simulink model "UZ_EnDat_be4_diffrework"  (R2023b)
settings: Solver=FixedStepDiscrete  StartTime=0  StopTime=0.002  RelTol=1e-3
model workspace (MAT data in the model file):
  Select = 0
libraries: hdlsllib x207, simulink x17, simulink_extras x3
(part 5 of 5)

== system UZ_EnDat_be4_diffrework/UZ_ENDAT/RESPONSESLICER5X/25BITSLICER/responseslicer2 ==
  DATA : Inport  OutDataTypeStr=uint64
  Bit Slice1 : hdlsllib/Logic and Bit Operations/Bit Slice  lidx=2  ridx=2
  Bit Slice3 : hdlsllib/Logic and Bit Operations/Bit Slice  lidx=31  ridx=27
  Bit Slice4 : hdlsllib/Logic and Bit Operations/Bit Slice  lidx=26  ridx=2
  Data Type Conversion1 : DataTypeConversion  OutDataTypeStr=boolean  SaturateOnIntegerOverflow=off  RndMeth=Floor
  Data Type Conversion3 : DataTypeConversion  OutDataTypeStr=uint8  SaturateOnIntegerOverflow=off  RndMeth=Floor
  Data Type Conversion4 : DataTypeConversion  OutDataTypeStr=uint32  SaturateOnIntegerOverflow=off  RndMeth=Floor
  Terminator : Terminator
  CRC : Outport  OutDataTypeStr=uint8
  payload : Outport  Port=2  OutDataTypeStr=uint32
  error : Outport  Port=3  OutDataTypeStr=boolean
  wires:
  DATA/1 -> Terminator/1, Bit Slice1/1, Bit Slice4/1, Bit Slice3/1
  Bit Slice3/1 -> Data Type Conversion3/1
  Bit Slice4/1 -> Data Type Conversion4/1
  Data Type Conversion3/1 -> CRC/1
  Data Type Conversion4/1 -> payload/1
  Bit Slice1/1 -> Data Type Conversion1/1
  Data Type Conversion1/1 -> error/1

== system UZ_EnDat_be4_diffrework/UZ_ENDAT/RESPONSESLICER5X/25BITSLICER/responseslicer3 ==
  DATA : Inport  OutDataTypeStr=uint64
  Bit Slice1 : hdlsllib/Logic and Bit Operations/Bit Slice  lidx=2  ridx=2
  Bit Slice3 : hdlsllib/Logic and Bit Operations/Bit Slice  lidx=31  ridx=27
  Bit Slice4 : hdlsllib/Logic and Bit Operations/Bit Slice  lidx=26  ridx=2
  Data Type Conversion1 : DataTypeConversion  OutDataTypeStr=boolean  SaturateOnIntegerOverflow=off  RndMeth=Floor
  Data Type Conversion3 : DataTypeConversion  OutDataTypeStr=uint8  SaturateOnIntegerOverflow=off  RndMeth=Floor
  Data Type Conversion4 : DataTypeConversion  OutDataTypeStr=uint32  SaturateOnIntegerOverflow=off  RndMeth=Floor
  Terminator : Terminator
  CRC : Outport  OutDataTypeStr=uint8
  payload : Outport  Port=2  OutDataTypeStr=uint32
  error : Outport  Port=3  OutDataTypeStr=boolean
  wires:
  DATA/1 -> Terminator/1, Bit Slice1/1, Bit Slice4/1, Bit Slice3/1
  Bit Slice3/1 -> Data Type Conversion3/1
  Bit Slice4/1 -> Data Type Conversion4/1
  Data Type Conversion3/1 -> CRC/1
  Data Type Conversion4/1 -> payload/1
  Bit Slice1/1 -> Data Type Conversion1/1
  Data Type Conversion1/1 -> error/1

== system UZ_EnDat_be4_diffrework/UZ_ENDAT/RESPONSESLICER5X/25BITSLICER/responseslicer4 ==
  DATA : Inport  OutDataTypeStr=uint64
  Bit Slice1 : hdlsllib/Logic and Bit Operations/Bit Slice  lidx=2  ridx=2
  Bit Slice3 : hdlsllib/Logic and Bit Operations/Bit Slice  lidx=31  ridx=27
  Bit Slice4 : hdlsllib/Logic and Bit Operations/Bit Slice  lidx=26  ridx=2
  Data Type Conversion1 : DataTypeConversion  OutDataTypeStr=boolean  SaturateOnIntegerOverflow=off  RndMeth=Floor
  Data Type Conversion3 : DataTypeConversion  OutDataTypeStr=uint8  SaturateOnIntegerOverflow=off  RndMeth=Floor
  Data Type Conversion4 : DataTypeConversion  OutDataTypeStr=uint32  SaturateOnIntegerOverflow=off  RndMeth=Floor
  Terminator : Terminator
  CRC : Outport  OutDataTypeStr=uint8
  payload : Outport  Port=2  OutDataTypeStr=uint32
  error : Outport  Port=3  OutDataTypeStr=boolean
  wires:
  DATA/1 -> Terminator/1, Bit Slice1/1, Bit Slice4/1, Bit Slice3/1
  Bit Slice3/1 -> Data Type Conversion3/1
  Bit Slice4/1 -> Data Type Conversion4/1
  Data Type Conversion3/1 -> CRC/1
  Data Type Conversion4/1 -> payload/1
  Bit Slice1/1 -> Data Type Conversion1/1
  Data Type Conversion1/1 -> error/1

== system UZ_EnDat_be4_diffrework/UZ_ENDAT/RESPONSESLICER5X/27BITSLICER/responseslicer ==
  DATA : Inport  OutDataTypeStr=uint64
  Bit Slice1 : hdlsllib/Logic and Bit Operations/Bit Slice  lidx=2  ridx=2
  Bit Slice3 : hdlsllib/Logic and Bit Operations/Bit Slice  lidx=33  ridx=29
  Bit Slice4 : hdlsllib/Logic and Bit Operations/Bit Slice  lidx=28  ridx=2
  Data Type Conversion1 : DataTypeConversion  OutDataTypeStr=boolean  SaturateOnIntegerOverflow=off  RndMeth=Floor
  Data Type Conversion3 : DataTypeConversion  OutDataTypeStr=uint8  SaturateOnIntegerOverflow=off  RndMeth=Floor
  Data Type Conversion4 : DataTypeConversion  OutDataTypeStr=uint32  SaturateOnIntegerOverflow=off  RndMeth=Floor
  Terminator : Terminator
  CRC : Outport  OutDataTypeStr=uint8
  payload : Outport  Port=2  OutDataTypeStr=uint32
  error : Outport  Port=3  OutDataTypeStr=boolean
  wires:
  DATA/1 -> Terminator/1, Bit Slice1/1, Bit Slice4/1, Bit Slice3/1
  Bit Slice3/1 -> Data Type Conversion3/1
  Bit Slice4/1 -> Data Type Conversion4/1
  Data Type Conversion3/1 -> CRC/1
  Data Type Conversion4/1 -> payload/1
  Bit Slice1/1 -> Data Type Conversion1/1
  Data Type Conversion1/1 -> error/1

== system UZ_EnDat_be4_diffrework/UZ_ENDAT/RESPONSESLICER5X/27BITSLICER/responseslicer1 ==
  DATA : Inport  OutDataTypeStr=uint64
  Bit Slice1 : hdlsllib/Logic and Bit Operations/Bit Slice  lidx=2  ridx=2
  Bit Slice3 : hdlsllib/Logic and Bit Operations/Bit Slice  lidx=33  ridx=29
  Bit Slice4 : hdlsllib/Logic and Bit Operations/Bit Slice  lidx=28  ridx=2
  Data Type Conversion1 : DataTypeConversion  OutDataTypeStr=boolean  SaturateOnIntegerOverflow=off  RndMeth=Floor
  Data Type Conversion3 : DataTypeConversion  OutDataTypeStr=uint8  SaturateOnIntegerOverflow=off  RndMeth=Floor
  Data Type Conversion4 : DataTypeConversion  OutDataTypeStr=uint32  SaturateOnIntegerOverflow=off  RndMeth=Floor
  Terminator : Terminator
  CRC : Outport  OutDataTypeStr=uint8
  payload : Outport  Port=2  OutDataTypeStr=uint32
  error : Outport  Port=3  OutDataTypeStr=boolean
  wires:
  DATA/1 -> Terminator/1, Bit Slice1/1, Bit Slice4/1, Bit Slice3/1
  Bit Slice3/1 -> Data Type Conversion3/1
  Bit Slice4/1 -> Data Type Conversion4/1
  Data Type Conversion3/1 -> CRC/1
  Data Type Conversion4/1 -> payload/1
  Bit Slice1/1 -> Data Type Conversion1/1
  Data Type Conversion1/1 -> error/1

== system UZ_EnDat_be4_diffrework/UZ_ENDAT/RESPONSESLICER5X/27BITSLICER/responseslicer2 ==
  DATA : Inport  OutDataTypeStr=uint64
  Bit Slice1 : hdlsllib/Logic and Bit Operations/Bit Slice  lidx=2  ridx=2
  Bit Slice3 : hdlsllib/Logic and Bit Operations/Bit Slice  lidx=33  ridx=29
  Bit Slice4 : hdlsllib/Logic and Bit Operations/Bit Slice  lidx=28  ridx=2
  Data Type Conversion1 : DataTypeConversion  OutDataTypeStr=boolean  SaturateOnIntegerOverflow=off  RndMeth=Floor
  Data Type Conversion3 : DataTypeConversion  OutDataTypeStr=uint8  SaturateOnIntegerOverflow=off  RndMeth=Floor
  Data Type Conversion4 : DataTypeConversion  OutDataTypeStr=uint32  SaturateOnIntegerOverflow=off  RndMeth=Floor
  Terminator : Terminator
  CRC : Outport  OutDataTypeStr=uint8
  payload : Outport  Port=2  OutDataTypeStr=uint32
  error : Outport  Port=3  OutDataTypeStr=boolean
  wires:
  DATA/1 -> Terminator/1, Bit Slice1/1, Bit Slice4/1, Bit Slice3/1
  Bit Slice3/1 -> Data Type Conversion3/1
  Bit Slice4/1 -> Data Type Conversion4/1
  Data Type Conversion3/1 -> CRC/1
  Data Type Conversion4/1 -> payload/1
  Bit Slice1/1 -> Data Type Conversion1/1
  Data Type Conversion1/1 -> error/1

== system UZ_EnDat_be4_diffrework/UZ_ENDAT/RESPONSESLICER5X/27BITSLICER/responseslicer3 ==
  DATA : Inport  OutDataTypeStr=uint64
  Bit Slice1 : hdlsllib/Logic and Bit Operations/Bit Slice  lidx=2  ridx=2
  Bit Slice3 : hdlsllib/Logic and Bit Operations/Bit Slice  lidx=33  ridx=29
  Bit Slice4 : hdlsllib/Logic and Bit Operations/Bit Slice  lidx=28  ridx=2
  Data Type Conversion1 : DataTypeConversion  OutDataTypeStr=boolean  SaturateOnIntegerOverflow=off  RndMeth=Floor
  Data Type Conversion3 : DataTypeConversion  OutDataTypeStr=uint8  SaturateOnIntegerOverflow=off  RndMeth=Floor
  Data Type Conversion4 : DataTypeConversion  OutDataTypeStr=uint32  SaturateOnIntegerOverflow=off  RndMeth=Floor
  Terminator : Terminator
  CRC : Outport  OutDataTypeStr=uint8
  payload : Outport  Port=2  OutDataTypeStr=uint32
  error : Outport  Port=3  OutDataTypeStr=boolean
  wires:
  DATA/1 -> Terminator/1, Bit Slice1/1, Bit Slice4/1, Bit Slice3/1
  Bit Slice3/1 -> Data Type Conversion3/1
  Bit Slice4/1 -> Data Type Conversion4/1
  Data Type Conversion3/1 -> CRC/1
  Data Type Conversion4/1 -> payload/1
  Bit Slice1/1 -> Data Type Conversion1/1
  Data Type Conversion1/1 -> error/1

== system UZ_EnDat_be4_diffrework/UZ_ENDAT/RESPONSESLICER5X/27BITSLICER/responseslicer4 ==
  DATA : Inport  OutDataTypeStr=uint64
  Bit Slice1 : hdlsllib/Logic and Bit Operations/Bit Slice  lidx=2  ridx=2
  Bit Slice3 : hdlsllib/Logic and Bit Operations/Bit Slice  lidx=33  ridx=29
  Bit Slice4 : hdlsllib/Logic and Bit Operations/Bit Slice  lidx=28  ridx=2
  Data Type Conversion1 : DataTypeConversion  OutDataTypeStr=boolean  SaturateOnIntegerOverflow=off  RndMeth=Floor
  Data Type Conversion3 : DataTypeConversion  OutDataTypeStr=uint8  SaturateOnIntegerOverflow=off  RndMeth=Floor
  Data Type Conversion4 : DataTypeConversion  OutDataTypeStr=uint32  SaturateOnIntegerOverflow=off  RndMeth=Floor
  Terminator : Terminator
  CRC : Outport  OutDataTypeStr=uint8
  payload : Outport  Port=2  OutDataTypeStr=uint32
  error : Outport  Port=3  OutDataTypeStr=boolean
  wires:
  DATA/1 -> Terminator/1, Bit Slice1/1, Bit Slice4/1, Bit Slice3/1
  Bit Slice3/1 -> Data Type Conversion3/1
  Bit Slice4/1 -> Data Type Conversion4/1
  Data Type Conversion3/1 -> CRC/1
  Data Type Conversion4/1 -> payload/1
  Bit Slice1/1 -> Data Type Conversion1/1
  Data Type Conversion1/1 -> error/1

== system UZ_EnDat_be4_diffrework/UZ_ENDAT/Subsystem/stalebootupfunction/CLKCNTERBOOTUP ==
  CLK : Inport
  CLK2CNT : Inport  Port=2
  ResetCNT : Inport  Port=3  OutDataTypeStr=boolean
  Delay1 : Delay  DelayLength=1
  Positional_Counter : Subsystem  TreatAsAtomicUnit=on
      settings: LibrarySourceBlock=|
      | hdlsllib/Ports &
      | Subsystems/Triggered
      | Subsystem
  SetZero32modified : Subsystem
  CNT : Outport
  wires:
  CLK2CNT/1 -> Positional_Counter/Trigger
  Delay1/1 -> Positional_Counter/1(valueout), CNT/1
  SetZero32modified/1(valueout) -> Delay1/1
  CLK/1 -> SetZero32modified/Trigger
  Positional_Counter/1(divider) -> SetZero32modified/1(valin)
  ResetCNT/1 -> SetZero32modified/2(setzero)

== system UZ_EnDat_be4_diffrework/UZ_ENDAT/Subsystem/stalebootupfunction/ManualDeserializere ==
  CLK : Inport
  SLOWCLCK : Inport  Port=2
  DATA : Inport  Port=3
  reset : Inport  Port=4
  14 : Inport  Port=5
  Constant3 : Constant  Value=0  OutDataTypeStr=boolean  SampleTime=-1
  Data Type Conversion : DataTypeConversion  OutMin=0  OutMax=1  OutDataTypeStr=fixdt(0,1)  SaturateOnIntegerOverflow=off  RndMeth=Floor
  Delay : Delay  DelayLength=1
  Delay1 : Delay  DelayLength=1
  Logical Operator : Logic  Operator=NOT  AllPortsSameDT=off  OutDataTypeStr=boolean
  Multiport Switch : MultiPortSwitch  Inputs=16  DataPortForDefault=Additional data port  DiagnosticForDefault=None  SaturateOnIntegerOverflow=off  InputSameDT=off
  Switch : Switch  Criteria=u2 ~= 0  SaturateOnIntegerOverflow=off  InputSameDT=off
  WORDTOBOOL : Subsystem  TreatAsAtomicUnit=on
  ramwatcher : Subsystem  TreatAsAtomicUnit=on
      settings: LibrarySourceBlock=|
      | hdlsllib/Ports &
      | Subsystems/Triggered
      | Subsystem
  valin : Outport
  wires:
  SLOWCLCK/1 -> Switch/1, Delay/1
  DATA/1 -> WORDTOBOOL/1(DATAIN)
  Multiport Switch/1 -> valin/1
  CLK/1 -> WORDTOBOOL/Trigger
  Delay1/1 -> ramwatcher/1(In1)
  Constant3/1 -> Multiport Switch/18
  reset/1 -> Logical Operator/1
  Logical Operator/1 -> Data Type Conversion/1
  Data Type Conversion/1 -> ramwatcher/2(In2)
  WORDTOBOOL/1(DATAOUT0) -> Multiport Switch/17
  WORDTOBOOL/2(DATAOUT1) -> Multiport Switch/16
  WORDTOBOOL/3(DATAOUT2) -> Multiport Switch/15
  WORDTOBOOL/4(DATAOUT3) -> Multiport Switch/14
  WORDTOBOOL/5(DATAOUT4) -> Multiport Switch/13
  WORDTOBOOL/6(DATAOUT5) -> Multiport Switch/12
  WORDTOBOOL/9(DATAOUT8) -> Multiport Switch/9
  WORDTOBOOL/10(DATAOUT9) -> Multiport Switch/8
  WORDTOBOOL/11(DATAOUT10) -> Multiport Switch/7
  WORDTOBOOL/12(DATAOUT11) -> Multiport Switch/6
  WORDTOBOOL/13(DATAOUT12) -> Multiport Switch/5
  WORDTOBOOL/14(DATAOUT13) -> Multiport Switch/4
  WORDTOBOOL/15(DATAOUT14) -> Multiport Switch/3
  WORDTOBOOL/16(DATAOUT15) -> Multiport Switch/2
  WORDTOBOOL/7(DATAOUT6) -> Multiport Switch/11
  WORDTOBOOL/8(DATAOUT7) -> Multiport Switch/10
  14/1 -> Switch/2
  ramwatcher/1(SEL) -> Multiport Switch/1, Delay1/1
  Switch/1 -> ramwatcher/Trigger
  Delay/1 -> Switch/3

== system UZ_EnDat_be4_diffrework/UZ_ENDAT/Subsystem/stalebootupfunction/OUTPUTCONTROLCONTINIOUS ==
  CLKCNT : Inport
  CLKS2DATAFLOWCHG : Inport  Port=2
  CLK2ENDOFTRANSMISSION : Inport  Port=3
  OPENCOM : Inport  Port=4
  Logical Operator : Logic  Operator=OR  AllPortsSameDT=off  OutDataTypeStr=boolean
  Logical Operator6 : Logic  Operator=NOT  Inputs=3  AllPortsSameDT=off  OutDataTypeStr=boolean
  Relational Operator : RelationalOperator  Operator=<=  OutDataTypeStr=boolean  InputSameDT=off
  Relational Operator1 : RelationalOperator  OutDataTypeStr=boolean  InputSameDT=off
  CLKOFF : Outport  OutDataTypeStr=boolean
  DATAINV : Outport  Port=2  OutDataTypeStr=boolean
  RESETCNT : Outport  Port=3  OutDataTypeStr=boolean
  wires:
  CLKCNT/1 -> Relational Operator1/1, Relational Operator/1
  CLKS2DATAFLOWCHG/1 -> Relational Operator/2
  Relational Operator/1 -> DATAINV/1
  CLK2ENDOFTRANSMISSION/1 -> Relational Operator1/2
  Relational Operator1/1 -> RESETCNT/1, Logical Operator/2
  Logical Operator/1 -> CLKOFF/1
  OPENCOM/1 -> Logical Operator6/1
  Logical Operator6/1 -> Logical Operator/1

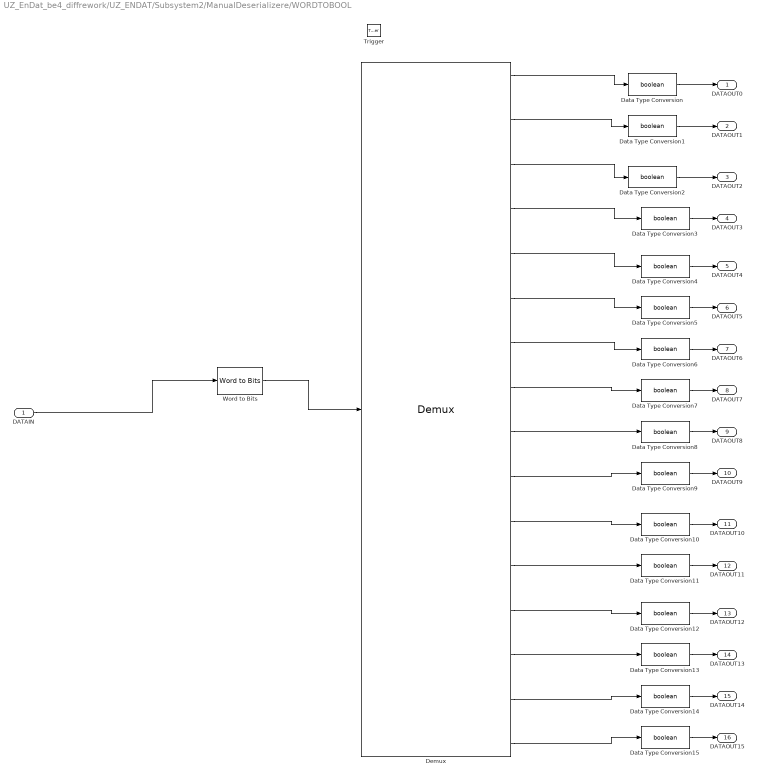
== system UZ_EnDat_be4_diffrework/UZ_ENDAT/Subsystem2/ManualDeserializere/WORDTOBOOL ==
  DATAIN : Inport
  Trigger : TriggerPort  TriggerType=falling  VariantControl=(inherit)  OutputDataType=int8  InitialTriggerSignalState=positive
  Data Type Conversion{,1..15} (16 alike) : DataTypeConversion  OutDataTypeStr=boolean  SaturateOnIntegerOverflow=off  RndMeth=Floor
  Demux : Demux  Outputs=16
  Word to Bits : hdlsllib/Logic and Bit Operations/Word to Bits  maxWordLength=16
  DATAOUT0 : Outport  InitialOutput=0
  DATAOUT1 : Outport  Port=2  InitialOutput=0
  DATAOUT2 : Outport  Port=3  InitialOutput=0
  DATAOUT3 : Outport  Port=4  InitialOutput=0
  DATAOUT4 : Outport  Port=5  InitialOutput=0
  DATAOUT5 : Outport  Port=6  InitialOutput=0
  DATAOUT6 : Outport  Port=7  InitialOutput=0
  DATAOUT7 : Outport  Port=8  InitialOutput=0
  DATAOUT8 : Outport  Port=9  InitialOutput=0
  DATAOUT9 : Outport  Port=10  InitialOutput=0
  DATAOUT10 : Outport  Port=11  InitialOutput=0
  DATAOUT11 : Outport  Port=12  InitialOutput=0
  DATAOUT12 : Outport  Port=13  InitialOutput=0
  DATAOUT13 : Outport  Port=14  InitialOutput=0
  DATAOUT14 : Outport  Port=15  InitialOutput=0
  DATAOUT15 : Outport  Port=16  InitialOutput=0
  wires:
  Demux/1 -> Data Type Conversion/1
  Demux/2 -> Data Type Conversion1/1
  Demux/4 -> Data Type Conversion3/1
  Demux/3 -> Data Type Conversion2/1
  Demux/6 -> Data Type Conversion5/1
  Demux/5 -> Data Type Conversion4/1
  Demux/8 -> Data Type Conversion7/1
  Demux/7 -> Data Type Conversion6/1
  Demux/10 -> Data Type Conversion9/1
  Demux/11 -> Data Type Conversion10/1
  Demux/12 -> Data Type Conversion11/1
  Demux/9 -> Data Type Conversion8/1
  Demux/13 -> Data Type Conversion12/1
  Demux/16 -> Data Type Conversion15/1
  Demux/14 -> Data Type Conversion13/1
  Demux/15 -> Data Type Conversion14/1
  Word to Bits/1 -> Demux/1
  Data Type Conversion/1 -> DATAOUT0/1
  Data Type Conversion1/1 -> DATAOUT1/1
  Data Type Conversion2/1 -> DATAOUT2/1
  Data Type Conversion3/1 -> DATAOUT3/1
  Data Type Conversion4/1 -> DATAOUT4/1
  Data Type Conversion5/1 -> DATAOUT5/1
  Data Type Conversion6/1 -> DATAOUT6/1
  Data Type Conversion7/1 -> DATAOUT7/1
  Data Type Conversion8/1 -> DATAOUT8/1
  Data Type Conversion9/1 -> DATAOUT9/1
  Data Type Conversion10/1 -> DATAOUT10/1
  Data Type Conversion11/1 -> DATAOUT11/1
  Data Type Conversion12/1 -> DATAOUT12/1
  Data Type Conversion13/1 -> DATAOUT13/1
  Data Type Conversion14/1 -> DATAOUT14/1
  Data Type Conversion15/1 -> DATAOUT15/1
  DATAIN/1 -> Word to Bits/1

== system UZ_EnDat_be4_diffrework/UZ_ENDAT/Subsystem2/ManualDeserializere/ramwatcher ==
  In1 : Inport  OutMin=0  OutMax=32000  OutDataTypeStr=uint16  LockScale=on
  reset : Inport  Port=2  OutMin=0  OutMax=1  OutDataTypeStr=boolean  LockScale=on
  Trigger : TriggerPort  VariantControl=(inherit)  OutputDataType=int8  InitialTriggerSignalState=zero
  Constant2 : Constant  Value=0  OutDataTypeStr=uint16  SampleTime=-1
  Increment Stored Integer : hdlsllib/Math Operations/Increment Stored Integer
  Index Vector1 : MultiPortSwitch  DataPortOrder=Zero-based contiguous  Inputs=2  zeroidx=on  SaturateOnIntegerOverflow=off  InputSameDT=off
  SEL : Outport  InitialOutput=0
  wires:
  In1/1 -> Increment Stored Integer/1
  Increment Stored Integer/1 -> Index Vector1/2
  Index Vector1/1 -> SEL/1
  Constant2/1 -> Index Vector1/3
  reset/1 -> Index Vector1/1

== system UZ_EnDat_be4_diffrework/UZ_ENDAT/responseslicer5/ENDAT23BITREVERSER/32BITREVERSE ==
  in : Inport
  16BITREVERSER : Subsystem
  16BITREVERSER1 : Subsystem
  Bit Concat : hdlsllib/Logic and Bit Operations/Bit Concat  numInputs=2
  Bit Slice : hdlsllib/Logic and Bit Operations/Bit Slice  lidx=15  ridx=0
  Bit Slice1 : hdlsllib/Logic and Bit Operations/Bit Slice  lidx=31  ridx=16
  out : Outport
  wires:
  in/1 -> Bit Slice1/1, Bit Slice/1
  16BITREVERSER/1(out) -> Bit Concat/1
  16BITREVERSER1/1(out) -> Bit Concat/2
  Bit Concat/1 -> out/1
  Bit Slice/1 -> 16BITREVERSER/1(in)
  Bit Slice1/1 -> 16BITREVERSER1/1(in)

== system UZ_EnDat_be4_diffrework/UZ_ENDAT/timingprovider/CLKCNTER_POSCNTR/Positional_Counter ==
  valueout : Inport  OutDataTypeStr=uint32
  Trigger : TriggerPort  VariantControl=(inherit)  InitialTriggerSignalState=zero
  Increment Stored Integer : hdlsllib/Math Operations/Increment Stored Integer
  divider : Outport  InitialOutput=0
  wires:
  valueout/1 -> Increment Stored Integer/1
  Increment Stored Integer/1 -> divider/1

== system UZ_EnDat_be4_diffrework/UZ_ENDAT/timingprovider/CLKCNTER_POSCNTR/SetZero32 ==
  valin : Inport
  setzero : Inport  Port=2  OutDataTypeStr=boolean
  Trigger : TriggerPort  TriggerType=either  VariantControl=(inherit)
  Constant1 : Constant  OutDataTypeStr=fixdt(0,1,0)  SampleTime=-1
  Constant2 : Constant  Value=0  OutDataTypeStr=fixdt(0,1,0)  SampleTime=-1
  Index Vector1 : MultiPortSwitch  DataPortOrder=Zero-based contiguous  Inputs=2  zeroidx=on  SaturateOnIntegerOverflow=off  InputSameDT=off
  Product : Product  OutDataTypeStr=uint32  RndMeth=Simplest  SaturateOnIntegerOverflow=on  LockScale=on
  valueout : Outport  InitialOutput=1  VectorParamsAs1DForOutWhenUnconnected=off
  wires:
  Index Vector1/1 -> Product/1
  valin/1 -> Product/2
  Product/1 -> valueout/1
  Constant1/1 -> Index Vector1/2
  Constant2/1 -> Index Vector1/3
  setzero/1 -> Index Vector1/1

== system UZ_EnDat_be4_diffrework/UZ_ENDAT/timingprovider/CLKCNTER_POSCNTR/SetZero32modified ==
  valin : Inport
  setzero : Inport  Port=2  OutDataTypeStr=boolean
  Trigger : TriggerPort  TriggerType=either  VariantControl=(inherit)
  Constant2 : Constant  Value=0  OutDataTypeStr=uint32  SampleTime=-1
  Index Vector1 : MultiPortSwitch  DataPortOrder=Zero-based contiguous  Inputs=2  zeroidx=on  SaturateOnIntegerOverflow=off  InputSameDT=off
  valueout : Outport  InitialOutput=1  VectorParamsAs1DForOutWhenUnconnected=off
  wires:
  valin/1 -> Index Vector1/2
  Index Vector1/1 -> valueout/1
  Constant2/1 -> Index Vector1/3
  setzero/1 -> Index Vector1/1

== system UZ_EnDat_be4_diffrework/UZ_ENDAT/timingprovider/CLKCNTER_POSCNTR/SetZero32modified1 ==
  valin : Inport
  setzero : Inport  Port=2  OutDataTypeStr=boolean
  Trigger : TriggerPort  TriggerType=either  VariantControl=(inherit)
  Constant2 : Constant  Value=0  OutDataTypeStr=uint32  SampleTime=-1
  Index Vector1 : MultiPortSwitch  DataPortOrder=Zero-based contiguous  Inputs=2  zeroidx=on  SaturateOnIntegerOverflow=off  InputSameDT=off
  valueout : Outport  InitialOutput=1  VectorParamsAs1DForOutWhenUnconnected=off
  wires:
  valin/1 -> Index Vector1/2
  Index Vector1/1 -> valueout/1
  Constant2/1 -> Index Vector1/3
  setzero/1 -> Index Vector1/1

== system UZ_EnDat_be4_diffrework/UZ_ENDAT/timingprovider/CLKCNTER_POSCNTR1/Positional_Counter ==
  valueout : Inport  OutDataTypeStr=uint32
  Trigger : TriggerPort  VariantControl=(inherit)  InitialTriggerSignalState=zero
  Increment Stored Integer : hdlsllib/Math Operations/Increment Stored Integer
  divider : Outport  InitialOutput=0
  wires:
  valueout/1 -> Increment Stored Integer/1
  Increment Stored Integer/1 -> divider/1

== system UZ_EnDat_be4_diffrework/UZ_ENDAT/timingprovider/CLKCNTER_POSCNTR1/SetZero32 ==
  valin : Inport
  setzero : Inport  Port=2  OutDataTypeStr=boolean
  Trigger : TriggerPort  TriggerType=either  VariantControl=(inherit)
  Constant1 : Constant  OutDataTypeStr=fixdt(0,1,0)  SampleTime=-1
  Constant2 : Constant  Value=0  OutDataTypeStr=fixdt(0,1,0)  SampleTime=-1
  Index Vector1 : MultiPortSwitch  DataPortOrder=Zero-based contiguous  Inputs=2  zeroidx=on  SaturateOnIntegerOverflow=off  InputSameDT=off
  Product : Product  OutDataTypeStr=uint32  RndMeth=Simplest  SaturateOnIntegerOverflow=on  LockScale=on
  valueout : Outport  InitialOutput=1  VectorParamsAs1DForOutWhenUnconnected=off
  wires:
  Index Vector1/1 -> Product/1
  valin/1 -> Product/2
  Product/1 -> valueout/1
  Constant1/1 -> Index Vector1/2
  Constant2/1 -> Index Vector1/3
  setzero/1 -> Index Vector1/1

== system UZ_EnDat_be4_diffrework/UZ_ENDAT/timingprovider/CLKCNTER_POSCNTR1/SetZero32modified ==
  valin : Inport
  setzero : Inport  Port=2  OutDataTypeStr=boolean
  Trigger : TriggerPort  TriggerType=either  VariantControl=(inherit)
  Constant2 : Constant  Value=0  OutDataTypeStr=uint32  SampleTime=-1
  Index Vector1 : MultiPortSwitch  DataPortOrder=Zero-based contiguous  Inputs=2  zeroidx=on  SaturateOnIntegerOverflow=off  InputSameDT=off
  valueout : Outport  InitialOutput=1  VectorParamsAs1DForOutWhenUnconnected=off
  wires:
  valin/1 -> Index Vector1/2
  Index Vector1/1 -> valueout/1
  Constant2/1 -> Index Vector1/3
  setzero/1 -> Index Vector1/1

== system UZ_EnDat_be4_diffrework/UZ_ENDAT/Subsystem/stalebootupfunction/CLKCNTERBOOTUP/Positional_Counter ==
  valueout : Inport  OutDataTypeStr=uint64
  Trigger : TriggerPort  VariantControl=(inherit)  InitialTriggerSignalState=zero
  Increment Stored Integer : hdlsllib/Math Operations/Increment Stored Integer
  divider : Outport  InitialOutput=0
  wires:
  valueout/1 -> Increment Stored Integer/1
  Increment Stored Integer/1 -> divider/1

== system UZ_EnDat_be4_diffrework/UZ_ENDAT/Subsystem/stalebootupfunction/CLKCNTERBOOTUP/SetZero32modified ==
  valin : Inport
  setzero : Inport  Port=2  OutDataTypeStr=boolean
  Trigger : TriggerPort  TriggerType=either  VariantControl=(inherit)
  Constant2 : Constant  Value=0  OutDataTypeStr=uint64  SampleTime=-1
  Index Vector1 : MultiPortSwitch  DataPortOrder=Zero-based contiguous  Inputs=2  zeroidx=on  OutDataTypeStr=uint64  SaturateOnIntegerOverflow=off  InputSameDT=off
  valueout : Outport  InitialOutput=1  VectorParamsAs1DForOutWhenUnconnected=off
  wires:
  valin/1 -> Index Vector1/2
  Index Vector1/1 -> valueout/1
  Constant2/1 -> Index Vector1/3
  setzero/1 -> Index Vector1/1

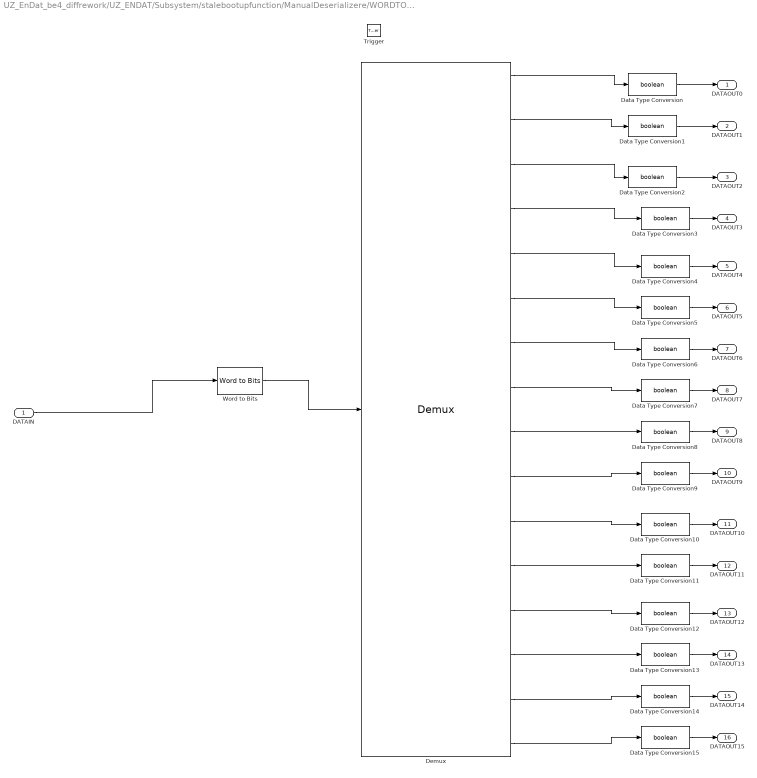
== system UZ_EnDat_be4_diffrework/UZ_ENDAT/Subsystem/stalebootupfunction/ManualDeserializere/WORDTOBOOL ==
  DATAIN : Inport
  Trigger : TriggerPort  TriggerType=falling  VariantControl=(inherit)  OutputDataType=int8  InitialTriggerSignalState=positive
  Data Type Conversion{,1..15} (16 alike) : DataTypeConversion  OutDataTypeStr=boolean  SaturateOnIntegerOverflow=off  RndMeth=Floor
  Demux : Demux  Outputs=16
  Word to Bits : hdlsllib/Logic and Bit Operations/Word to Bits  maxWordLength=16
  DATAOUT0 : Outport  InitialOutput=0
  DATAOUT1 : Outport  Port=2  InitialOutput=0
  DATAOUT2 : Outport  Port=3  InitialOutput=0
  DATAOUT3 : Outport  Port=4  InitialOutput=0
  DATAOUT4 : Outport  Port=5  InitialOutput=0
  DATAOUT5 : Outport  Port=6  InitialOutput=0
  DATAOUT6 : Outport  Port=7  InitialOutput=0
  DATAOUT7 : Outport  Port=8  InitialOutput=0
  DATAOUT8 : Outport  Port=9  InitialOutput=0
  DATAOUT9 : Outport  Port=10  InitialOutput=0
  DATAOUT10 : Outport  Port=11  InitialOutput=0
  DATAOUT11 : Outport  Port=12  InitialOutput=0
  DATAOUT12 : Outport  Port=13  InitialOutput=0
  DATAOUT13 : Outport  Port=14  InitialOutput=0
  DATAOUT14 : Outport  Port=15  InitialOutput=0
  DATAOUT15 : Outport  Port=16  InitialOutput=0
  wires:
  Demux/1 -> Data Type Conversion/1
  Demux/2 -> Data Type Conversion1/1
  Demux/4 -> Data Type Conversion3/1
  Demux/3 -> Data Type Conversion2/1
  Demux/6 -> Data Type Conversion5/1
  Demux/5 -> Data Type Conversion4/1
  Demux/8 -> Data Type Conversion7/1
  Demux/7 -> Data Type Conversion6/1
  Demux/10 -> Data Type Conversion9/1
  Demux/11 -> Data Type Conversion10/1
  Demux/12 -> Data Type Conversion11/1
  Demux/9 -> Data Type Conversion8/1
  Demux/13 -> Data Type Conversion12/1
  Demux/16 -> Data Type Conversion15/1
  Demux/14 -> Data Type Conversion13/1
  Demux/15 -> Data Type Conversion14/1
  Word to Bits/1 -> Demux/1
  Data Type Conversion/1 -> DATAOUT0/1
  Data Type Conversion1/1 -> DATAOUT1/1
  Data Type Conversion2/1 -> DATAOUT2/1
  Data Type Conversion3/1 -> DATAOUT3/1
  Data Type Conversion4/1 -> DATAOUT4/1
  Data Type Conversion5/1 -> DATAOUT5/1
  Data Type Conversion6/1 -> DATAOUT6/1
  Data Type Conversion7/1 -> DATAOUT7/1
  Data Type Conversion8/1 -> DATAOUT8/1
  Data Type Conversion9/1 -> DATAOUT9/1
  Data Type Conversion10/1 -> DATAOUT10/1
  Data Type Conversion11/1 -> DATAOUT11/1
  Data Type Conversion12/1 -> DATAOUT12/1
  Data Type Conversion13/1 -> DATAOUT13/1
  Data Type Conversion14/1 -> DATAOUT14/1
  Data Type Conversion15/1 -> DATAOUT15/1
  DATAIN/1 -> Word to Bits/1

== system UZ_EnDat_be4_diffrework/UZ_ENDAT/Subsystem/stalebootupfunction/ManualDeserializere/ramwatcher ==
  In1 : Inport  OutMin=0  OutMax=32000  OutDataTypeStr=uint16  LockScale=on
  In2 : Inport  Port=2  OutMin=0  OutMax=1  OutDataTypeStr=fixdt(0,1)  LockScale=on
  Trigger : TriggerPort  VariantControl=(inherit)  OutputDataType=int8  InitialTriggerSignalState=zero
  Increment Stored Integer : hdlsllib/Math Operations/Increment Stored Integer
  Product : Product  RndMeth=Simplest
  SEL : Outport  InitialOutput=0
  wires:
  In1/1 -> Increment Stored Integer/1
  Increment Stored Integer/1 -> Product/1
  Product/1 -> SEL/1
  In2/1 -> Product/2

== system UZ_EnDat_be4_diffrework/UZ_ENDAT/responseslicer5/ENDAT23BITREVERSER/32BITREVERSE/16BITREVERSER ==
  in : Inport
  Bit Concat : hdlsllib/Logic and Bit Operations/Bit Concat  numInputs=4
  Bit Slice : hdlsllib/Logic and Bit Operations/Bit Slice  lidx=3  ridx=0
  Bit Slice1 : hdlsllib/Logic and Bit Operations/Bit Slice  lidx=7  ridx=4
  Bit Slice2 : hdlsllib/Logic and Bit Operations/Bit Slice  lidx=11  ridx=8
  Bit Slice3 : hdlsllib/Logic and Bit Operations/Bit Slice  lidx=15  ridx=12
  out : Outport
  wires:
  in/1 -> Bit Slice/1, Bit Slice3/1, Bit Slice2/1, Bit Slice1/1
  Bit Slice1/1 -> Bit Concat/2
  Bit Slice/1 -> Bit Concat/1
  Bit Slice2/1 -> Bit Concat/3
  Bit Slice3/1 -> Bit Concat/4
  Bit Concat/1 -> out/1

== system UZ_EnDat_be4_diffrework/UZ_ENDAT/responseslicer5/ENDAT23BITREVERSER/32BITREVERSE/16BITREVERSER1 ==
  in : Inport
  Bit Concat : hdlsllib/Logic and Bit Operations/Bit Concat  numInputs=4
  Bit Slice : hdlsllib/Logic and Bit Operations/Bit Slice  lidx=3  ridx=0
  Bit Slice1 : hdlsllib/Logic and Bit Operations/Bit Slice  lidx=7  ridx=4
  Bit Slice2 : hdlsllib/Logic and Bit Operations/Bit Slice  lidx=11  ridx=8
  Bit Slice3 : hdlsllib/Logic and Bit Operations/Bit Slice  lidx=15  ridx=12
  out : Outport
  wires:
  in/1 -> Bit Slice/1, Bit Slice3/1, Bit Slice2/1, Bit Slice1/1
  Bit Slice1/1 -> Bit Concat/2
  Bit Slice/1 -> Bit Concat/1
  Bit Slice2/1 -> Bit Concat/3
  Bit Slice3/1 -> Bit Concat/4
  Bit Concat/1 -> out/1
